simulink model "plus_generator_edge_trigger1"  (R2018a)
settings: Solver=VariableStepAuto  StartTime=0.0  StopTime=10.0  RelTol=1e-3
settings Model: Creator=86188  LastModifiedBy=86188

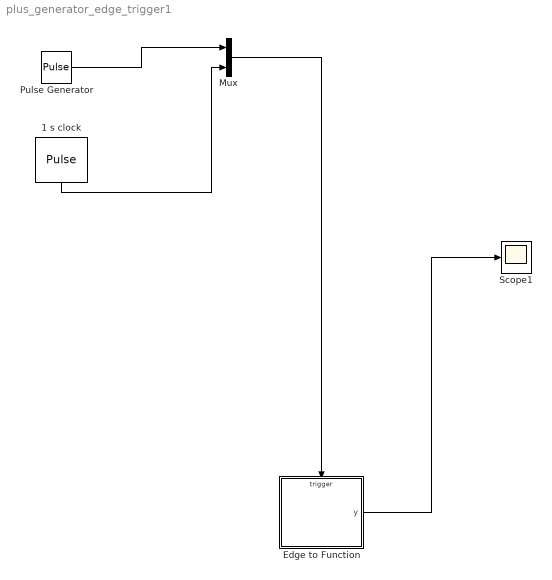
== system plus_generator_edge_trigger1 ==
  1 s clock : DiscretePulseGenerator  SampleTime=2
  "Edge to Function " : Stateflow chart  TreatAsAtomicUnit=on
  Mux : Mux  Inputs=2
  Pulse Generator : DiscretePulseGenerator  PulseType=Time based  Period=10  PulseWidth=5
  Scope1 : Scope
  wires:
  1 s clock/1 -> Mux/2
  "Edge to Function "/1(y) -> Scope1/1
  Pulse Generator/1 -> Mux/1
  Mux/1 -> "Edge to Function "/Trigger

== stateflow chart plus_generator_edge_trigger1/Edge to Function  ==
  (default) -> (junction 2) : {y=y+1;}
  data: y output int32 =0
  events: edge input RISING_EDGE_EVENT; event input FALLING_EDGE_EVENT
